simulink model "BioreactorTempTrialREADY"  (R2025b)
settings: Solver=FixedStepAuto  StartTime=0.0  StopTime=500  FixedStep=0.1  MaxStep=0.1  MinStep=0.1  RelTol=1e-3
libraries: slpidlib x1
settings Model: Creator=matth  LastModifiedBy=Lachy
settings SolverCC: InitialStep=0.1  ZeroCrossAlgorithm=Adaptive  AlgebraicLoopSolver=TrustRegion
settings DebuggingCC: IgnoredZcDiagnostic=none  UnconnectedInputMsg=warning  UnconnectedOutputMsg=warning  UnconnectedLineMsg=warning
settings ModelReferenceCC: EnableRefExpFcnMdlSchedulingChecks=on
settings RTWCC: GPUComputeCapability=3.5

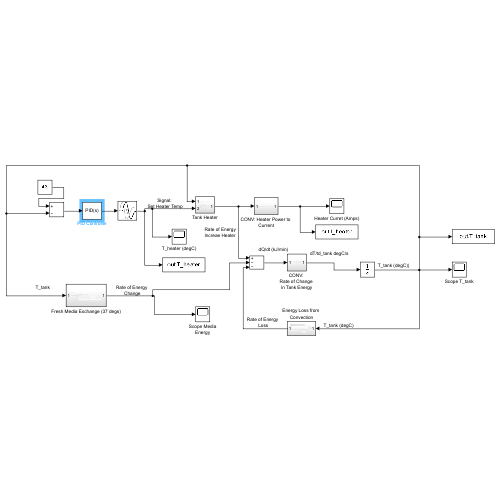
[thumbnail: Simulink's stored preview of the top-level diagram]
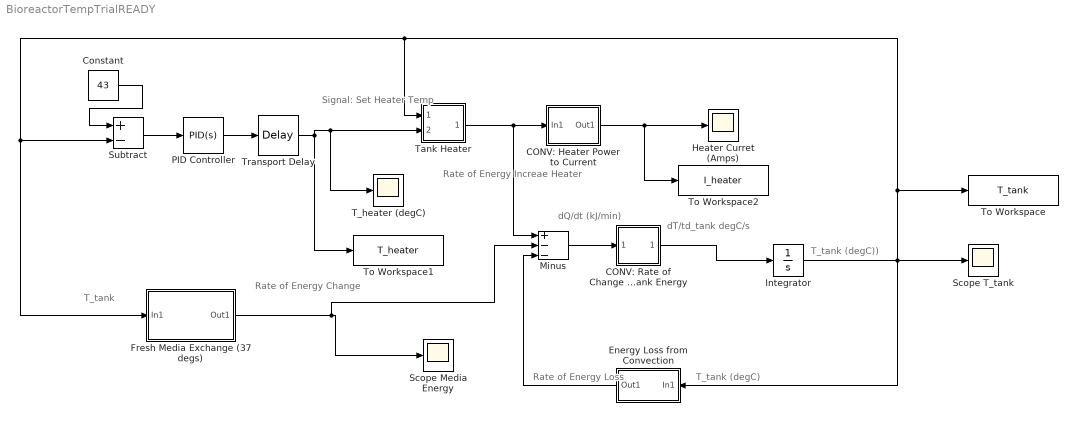
== system BioreactorTempTrialREADY ==
  note: Signal:
      | Set Heater Temp
  note: Rate of Energy
      | Loss
  note: T_tank (degC))
  note: Rate of Energy
      | Increae Heater
  note: dT/td_tank degC/s
  note: dQ/dt (kJ/min)
  note: T_tank (degC)
  note: Rate of Energy
      | Change
  note: T_tank
  "CONV: Rate of Change in Tank Energy " : Subsystem
  CONV: Heater Power to Current : Subsystem
  Constant : Constant  Value=43
  Energy Loss from Convection : Subsystem
  Fresh Media Exchange (37 degs) : Subsystem
  Heater Curret (Amps) : Scope
      settings: ActiveDisplayYMinimum=0  ActiveDisplayYMaximum=55  DataLoggingMaxPoints=4500
  Integrator : Integrator  InitialCondition=43
  Minus : Sum  Inputs=+--
  PID Controller : slpidlib/PID Controller  Controller=PID  Form=Parallel  TimeDomain=Continuous-time  UseExternalTs=off  SampleTime=-1  IntegratorMethod=Forward Euler  FilterMethod=Forward Euler  ControllerParametersSource=internal  P=1  I=1  UseKiTs=off  D=0  UseExternalDerivativeSource=off  N=100  UseFilter=on  TunerSelectOption=Transfer Function Based (PID Tuner App)  InitialConditionSource=internal  InitialConditionForIntegrator=0  InitialConditionForFilter=0  DifferentiatorICPrevScaledInput=0  ExternalReset=none  TrackingMode=off  Kt=1  LimitOutput=off  SatLimitsSource=internal  UpperSaturationLimit=inf  LowerSaturationLimit=-inf  LinearizeAsGain=on  AntiWindupMode=none  Kb=1  LimitIntegrator=off  UpperIntegratorSaturationLimit=inf  LowerIntegratorSaturationLimit=-inf  POutMin=[]  POutMax=[]  IOutMin=[]  IOutMax=[]  DOutMin=[]  DOutMax=[]  NOutMin=[]  NOutMax=[]  SumOutMin=[]  SumOutMax=[]  SaturationOutMin=[]  SaturationOutMax=[]  PParamMin=[]  PParamMax=[]  IParamMin=[]  IParamMax=[]  DParamMin=[]  DParamMax=[]  NParamMin=[]  NParamMax=[]  KbParamMin=[]  KbParamMax=[]  KtParamMin=[]  KtParamMax=[]  KbOutMin=[]  KbOutMax=[]  KtOutMin=[]  KtOutMax=[]  IntegratorOutMin=[]  IntegratorOutMax=[]  FilterOutMin=[]  FilterOutMax=[]  SumI1OutMin=[]  SumI1OutMax=[]  SumI2OutMin=[]  SumI2OutMax=[]  SumI3OutMin=[]  SumI3OutMax=[]  SumI4OutMin=[]  SumI4OutMax=[]  SumDOutMin=[]  SumDOutMax=[]  DifferentiatorOutMin=[]  DifferentiatorOutMax=[]  FilterDiffOutCoefMin=[]  FilterDiffOutCoefMax=[]  ReciprocalOutMin=[]  ReciprocalOutMax=[]  SumDenOutMin=[]  SumDenOutMax=[]  SumNumOutMin=[]  SumNumOutMax=[]  DivideOutMin=[]  DivideOutMax=[]  UdiffTsProdOutMin=[]  UdiffTsProdOutMax=[]  NTsProdOutMin=[]  NTsProdOutMax=[]  UintegralTsProdOutMin=[]  UintegralTsProdOutMax=[]  UngainTsProdOutMin=[]  UngainTsProdOutMax=[]  ClampingZeroOutDataTypeStr=Inherit: Inherit via back propagation  ClampingZeroOutMin=[]  ClampingZeroOutMax=[]  FilterDenConstantOutDataTypeStr=Inherit: Inherit via back propagation  FilterDenConstantOutMin=[]  FilterDenConstantOutMax=[]  PCopyOutDataTypeStr=Inherit: Inherit via back propagation  PCopyOutMin=[]  PCopyOutMax=[]  NCopyOutDataTypeStr=Inherit: Inherit via back propagation  NCopyOutMin=[]  NCopyOutMax=[]  IntegratorContinuousStateAttributes=''  IntegratorStateMustResolveToSignalObject=off  IntegratorRTWStateStorageClass=Auto  FilterContinuousStateAttributes=''  FilterStateMustResolveToSignalObject=off  FilterRTWStateStorageClass=Auto  ParallelPVariant=InternalParameters  IdealPVariant=Disabled  IVariant=InternalParameters  DVariant=InternalParameters  IntegratorVariant=Continuous  SatVariant=Disabled  AWVariant=Passthrough  PCopyVariant=Disabled  TRVariant=Disabled  FdbkBlocksVariant=Forward  IdealPFdbkVariant=Disabled  SatFdbkVariant=Disabled  DerivativeFilterVariant=ContFilter  NVariant=InternalParameters  NCopyVariant=Disabled  FilterICVariant=InternalICsFilter  IntegratorICVariant=InternalICs  ExternalResetVariant=Disabled  TRSumVariant=Passthrough  SumFdbkVariant=Disabled  SumVariant=Sum_PID  TsampFilterVariant=InternalTs  TsampNgainVariant=Passthrough  TsampIntegralVariant=Disabled_SignalSpec  ExternalSaturationOutDataTypeStr=Inherit: Same as second input  DerivativeSourceVariant=ErrorSignal  PreIntVariant=InternalPreInt
  Scope Media Energy : Scope
      settings: ActiveDisplayYMinimum=-235.34999999999997  ActiveDisplayYMaximum=2118.15  DataLoggingVariableName=ScopeData2
  Scope T_tank : Scope
      settings: ActiveDisplayYMinimum=40.753814322297487  ActiveDisplayYMaximum=49.743911854299355  DataLoggingMaxPoints=4500
  Subtract : Sum  Inputs=+-
  T_heater (degC) : Scope
      settings: ActiveDisplayYMinimum=-1.01167  ActiveDisplayYMaximum=77.43833  DataLoggingMaxPoints=4500  DataLoggingVariableName=ScopeData2
  Tank Heater : Subsystem
  To Workspace : ToWorkspace  VariableName=T_tank  SampleTime=-1
  To Workspace1 : ToWorkspace  VariableName=T_heater  SampleTime=-1
  To Workspace2 : ToWorkspace  VariableName=I_heater  SampleTime=-1
  Transport Delay : TransportDelay  DelayTime=0
  wires:
  Integrator/1 -> Subtract/2, Fresh Media Exchange (37 degs)/1(In1), Tank Heater/1(In1), To Workspace/1, Scope T_tank/1, Energy Loss from Convection/1(In1)
  PID Controller/1 -> Transport Delay/1
  Fresh Media Exchange (37 degs)/1(Out1) -> Minus/2, Scope Media Energy/1
  Tank Heater/1(Out1) -> Minus/1, CONV: Heater Power to Current/1(In1)
  CONV: Heater Power to Current/1(Out1) -> Heater Curret (Amps)/1, To Workspace2/1
  Minus/1 -> "CONV: Rate of Change in Tank Energy "/1(In1)
  "CONV: Rate of Change in Tank Energy "/1(Out1) -> Integrator/1
  Energy Loss from Convection/1(Out1) -> Minus/3
  Transport Delay/1 -> Tank Heater/2(In2), T_heater (degC)/1, To Workspace1/1
  Subtract/1 -> PID Controller/1
  Constant/1 -> Subtract/1

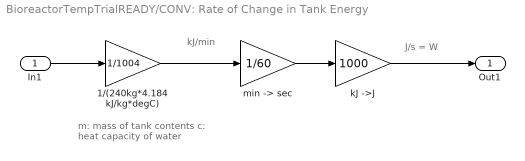
== system BioreactorTempTrialREADY/CONV: Rate of Change in Tank Energy  ==
  note: J/s = W
  note: kJ/min
  note: m: mass of tank contents
      | c: heat capacity of water
  In1 : Inport
  1/(240kg*4.184 kJ/kg*degC) : Gain  Gain=1/1004
  kJ ->J : Gain  Gain=1000
  "min -> sec" : Gain  Gain=1/60
  Out1 : Outport
  wires:
  In1/1 -> 1/(240kg*4.184 kJ/kg*degC)/1
  1/(240kg*4.184 kJ/kg*degC)/1 -> "min -> sec"/1
  "min -> sec"/1 -> kJ ->J/1
  kJ ->J/1 -> Out1/1

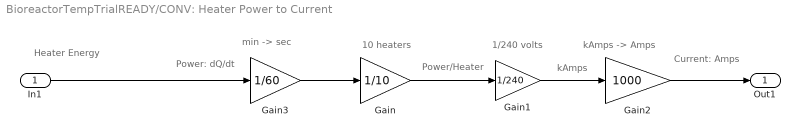
== system BioreactorTempTrialREADY/CONV: Heater Power to Current ==
  note: min -> sec
  note: Heater Energy
  note: Current: Amps
  note: kAmps -> Amps
  note: kAmps
  note: 1/240 volts
  note: Power/Heater
  note: 10 heaters
  note: Power: dQ/dt
  In1 : Inport
  Gain : Gain  Gain=1/10
  Gain1 : Gain  Gain=1/240
  Gain2 : Gain  Gain=1000
  Gain3 : Gain  Gain=1/60
  Out1 : Outport
  wires:
  In1/1 -> Gain3/1
  Gain/1 -> Gain1/1
  Gain1/1 -> Gain2/1
  Gain2/1 -> Out1/1
  Gain3/1 -> Gain/1

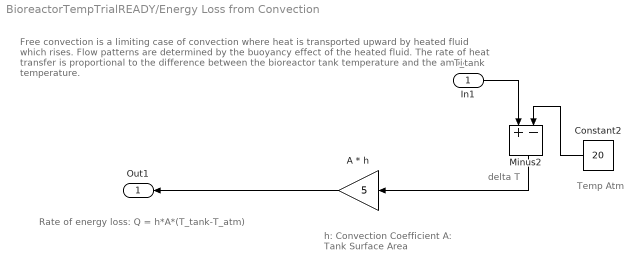
== system BioreactorTempTrialREADY/Energy Loss from Convection ==
  note: h: Convection Coefficient
      | A: Tank Surface Area
  note: Free convection is a limiting case of convection where heat is transported upward by heated fluid which rises. Flow patterns are determined by the buoyancy effect of the heated fluid. The rate of heat transfer is proportional to the difference between the bioreactor tank temperature and the ambient temperature.
  note: Rate of energy loss: Q = h*A*(T_tank-T_atm)
  note: T_tank
  note: delta T
  note: Temp Atm
  In1 : Inport
  A * h : Gain  Gain=5
  Constant2 : Constant  Value=20
  Minus2 : Sum  Inputs=+-
  Out1 : Outport
  wires:
  Minus2/1 -> A * h/1
  Constant2/1 -> Minus2/2
  In1/1 -> Minus2/1
  A * h/1 -> Out1/1

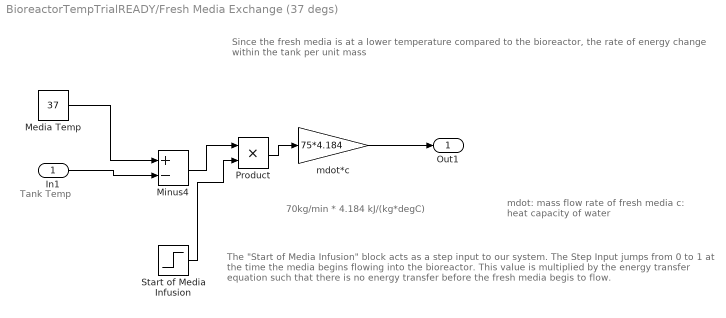
== system BioreactorTempTrialREADY/Fresh Media Exchange (37 degs) ==
  note: Since the fresh media is at a lower temperature compared to the bioreactor, the rate of energy change within the tank per unit mass
  note: The "Start of Media Infusion" block acts as a step input to our system. The Step Input jumps from 0 to 1 at the time the media begins flowing into the bioreactor. This value is multiplied by the energy transfer equation such that there is no energy transfer before the fresh media begis to flow.
  note: mdot: mass flow rate of fresh media
      | c: heat capacity of water
  note: Tank Temp
  note: 70kg/min * 4.184 kJ/(kg*degC)
  In1 : Inport
  Media Temp : Constant  Value=37
  Minus4 : Sum  Inputs=+-
  Product : Product
  Start of Media Infusion : Step  Time=180  After=-1  SampleTime=0
  mdot*c : Gain  Gain=75*4.184
  Out1 : Outport
  wires:
  Minus4/1 -> Product/1
  Start of Media Infusion/1 -> Product/2
  Media Temp/1 -> Minus4/1
  Product/1 -> mdot*c/1
  mdot*c/1 -> Out1/1
  In1/1 -> Minus4/2

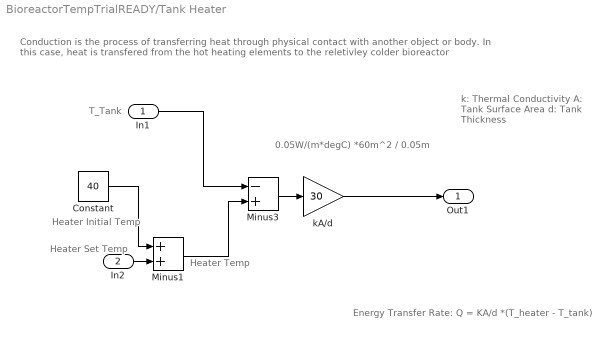
== system BioreactorTempTrialREADY/Tank Heater ==
  note: Heater Temp
  note: Heater Initial Temp
  note: Energy Transfer Rate: Q = KA/d *(T_heater - T_tank)
  note: Conduction is the process of transferring heat through physical contact with another object or body.
      | In this case, heat is transfered from the hot heating elements to the reletivley colder bioreactor
  note: T_Tank
  note: Heater Set
      | Temp
  note: k: Thermal Conductivity
      | A: Tank Surface Area
      | d: Tank Thickness
  note: 0.05W/(m*degC) *60m^2 / 0.05m
  In1 : Inport
  In2 : Inport  Port=2
  Constant : Constant  Value=40
  Minus1 : Sum
  Minus3 : Sum  Inputs=-+
  kA/d : Gain  Gain=30
  Out1 : Outport
  wires:
  Minus3/1 -> kA/d/1
  In1/1 -> Minus3/1
  kA/d/1 -> Out1/1
  In2/1 -> Minus1/2
  Minus1/1 -> Minus3/2
  Constant/1 -> Minus1/1
